simulink model "ESTS_REV_VWhlFild_test"  (R2023b)
settings: Solver=VariableStepAuto  StartTime=0.0  StopTime=10.0  RelTol=1e-3
libraries: ESTS_REV_VWhlFild x1
settings Model: Creator=blatak  LastModifiedBy=blatak

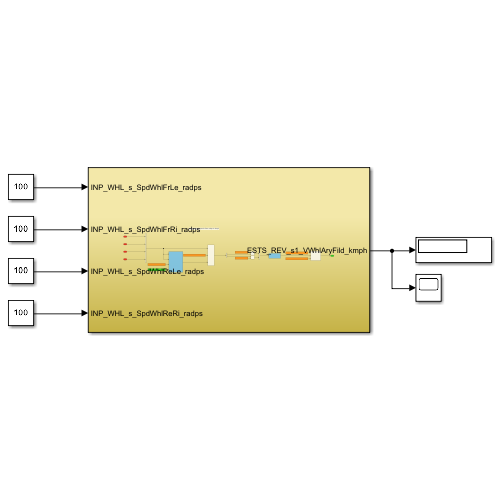
[thumbnail: Simulink's stored preview of the top-level diagram]
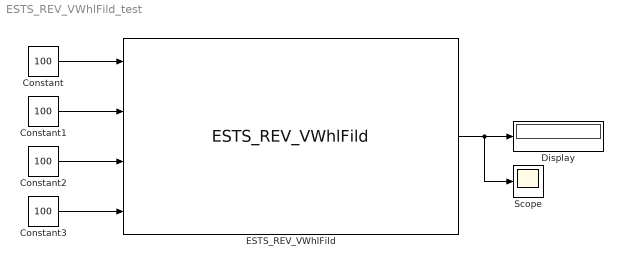
== system ESTS_REV_VWhlFild_test ==
  Constant{,1..3} (4 alike) : Constant  Value=100  OutDataTypeStr=single
  Display : Display
  ESTS_REV_VWhlFild : ESTS_REV_VWhlFild/ESTS_REV_VWhlFild  SystemSampleTime=-1  VariantActivationTime=update diagram  AllowFlexibleInterface=on  Latency=0  AutoFrameSizeCalculation=off
  Scope : Scope
  wires:
  Constant/1 -> ESTS_REV_VWhlFild/1
  Constant1/1 -> ESTS_REV_VWhlFild/2
  Constant2/1 -> ESTS_REV_VWhlFild/3
  Constant3/1 -> ESTS_REV_VWhlFild/4
  ESTS_REV_VWhlFild/1 -> Scope/1, Display/1
